simulink model "Ejercicio30"  (R2023b)
settings: Solver=VariableStepAuto  StartTime=0.0  StopTime=10  RelTol=1e-3
settings Model: Creator=mende  LastModifiedBy=mende

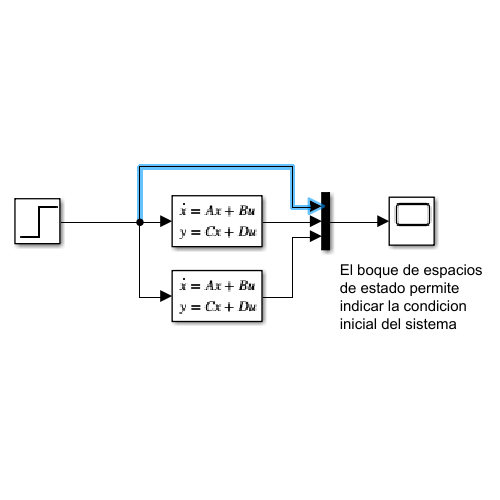
[thumbnail: Simulink's stored preview of the top-level diagram]
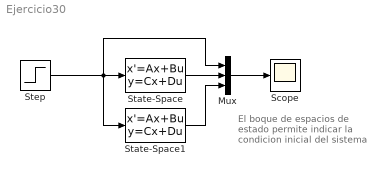
== system Ejercicio30 ==
  note: El boque de espacios de estado permite indicar la condicion inicial del sistema
  Mux : Mux  Inputs=3
  Scope : Scope
  State-Space : StateSpace  A=[-3 1 0;-2 0 0; 1 0 0]  B=[2; 4; 1]  C=[1 0 0]  D=0  InitialCondition=0.5  ParameterTunability=Optimized
  State-Space1 : StateSpace  A=[-3 1 0;-2 0 0; 1 0 0]  B=[2; 4; 1]  C=[1 0 0]  D=0  InitialCondition=0  ParameterTunability=Optimized
  Step : Step  Time=0.05  SampleTime=0  ZeroCross=off
  wires:
  State-Space/1 -> Mux/2
  Mux/1 -> Scope/1
  Step/1 -> Mux/1, State-Space/1, State-Space1/1
  State-Space1/1 -> Mux/3
